simulink model "cstr_sim_modified"  (R2017a)
settings: Solver=ode45  StartTime=0.0  StopTime=10  RelTol=1e-3  EnableMultiTasking=on
StopFcn:
  | plot_reactor
settings Model: Creator=tsladeche  LastModifiedBy=ljxia_000
settings DataIOCC: LimitDataPoints=on  SaveFormat=Array  SignalLoggingSaveFormat=ModelDataLogs
settings OptimizationCC: ExpressionDepthLimit=2147483647  LifeSpan=inf
settings DebuggingCC: UnderspecifiedInitializationDetection=Classic  MergeDetectMultiDrivingBlocksExec=none  SolverPrmCheckMsg=warning  FcnCallInpInsideContextMsg=warning  StateNameClashWarn=warning  SFUnexpectedBacktrackingDiag=warning  SFNoUnconditionalDefaultTransitionDiag=warning  SFExecutionAtInitializationDiag=none
settings HardwareCC: ProdBitPerPointer=32  ProdBitPerSizeT=32  ProdBitPerPtrDiffT=32  ProdLargestAtomicFloat=None  ProdIntDivRoundTo=Undefined  ProdEndianess=Unspecified  ProdWordSize=32  ProdHWDeviceType=32-bit Generic
settings ModelReferenceCC: PropagateSignalLabelsOutOfModel=off
settings GRTTargetCC: TargetLangStandard=C89/C90 (ANSI)  GeneratePreprocessorConditionals=Disable all  CombineOutputUpdateFcns=off  GRTInterface=on
settings ConfigComp: CovMetricSettings=dw  CovHtmlReporting=on  CovSaveCumulativeToWorkspaceVar=on  CovSaveSingleToWorkspaceVar=on  CovExternalEMLEnable=off

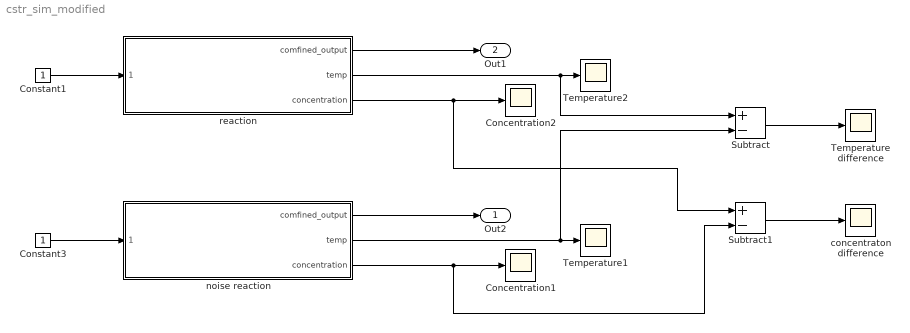
== system cstr_sim_modified ==
  Concentration1 : Scope
  Concentration2 : Scope
  Constant1 : Constant  SampleTime=0.01
  Constant3 : Constant  SampleTime=0.01
  Subtract : Sum  Inputs=+-
  Subtract1 : Sum  Inputs=+-
  Temperature difference : Scope
  Temperature1 : Scope
  Temperature2 : Scope
  concentraton difference : Scope
  noise reaction : Subsystem
  reaction : Subsystem
  Out2 : Outport
  Out1 : Outport  Port=2
  wires:
  noise reaction/1(comfined_output) -> Out2/1
  noise reaction/2(temp) -> Subtract/2, Temperature1/1
  noise reaction/3(concentration) -> Subtract1/2, Concentration1/1
  Constant3/1 -> noise reaction/1(1)
  reaction/1(comfined_output) -> Out1/1
  reaction/3(concentration) -> Subtract1/1, Concentration2/1
  Constant1/1 -> reaction/1(1)
  reaction/2(temp) -> Subtract/1, Temperature2/1
  Subtract/1 -> Temperature difference/1
  Subtract1/1 -> concentraton difference/1

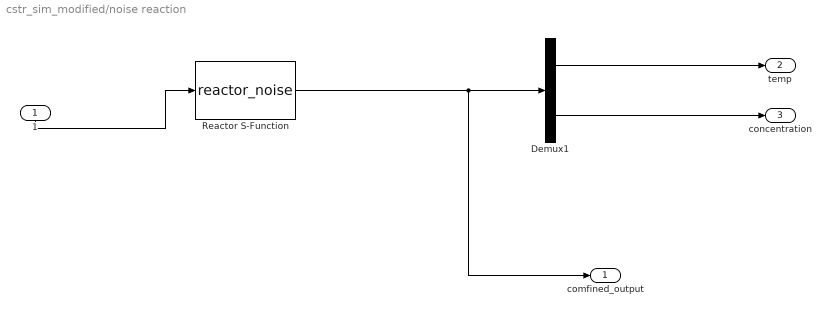
== system cstr_sim_modified/noise reaction ==
  1 : Inport
  Demux1 : Demux  Outputs=2
  Reactor S-Function : S-Function  FunctionName=reactor_noise  SFunctionDeploymentMode=off  EnableBusSupport=off
  comfined_output : Outport
  temp : Outport  Port=2
  concentration : Outport  Port=3
  wires:
  Demux1/2 -> concentration/1
  Reactor S-Function/1 -> comfined_output/1, Demux1/1
  Demux1/1 -> temp/1
  1/1 -> Reactor S-Function/1

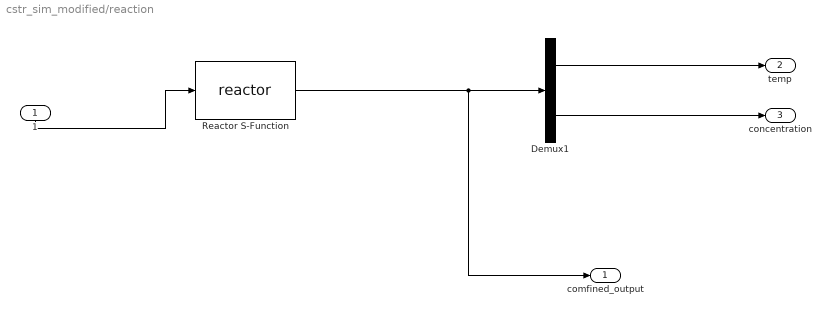
== system cstr_sim_modified/reaction ==
  1 : Inport
  Demux1 : Demux  Outputs=2
  "Reactor S-Function " : S-Function  FunctionName=reactor  SFunctionDeploymentMode=off  EnableBusSupport=off
  comfined_output : Outport
  temp : Outport  Port=2
  concentration : Outport  Port=3
  wires:
  Demux1/2 -> concentration/1
  "Reactor S-Function "/1 -> comfined_output/1, Demux1/1
  Demux1/1 -> temp/1
  1/1 -> "Reactor S-Function "/1
